simulink model "JFBH"  (Simulink 5.0)
settings: Solver=ode4  StartTime=0.0  StopTime=1  FixedStep=0.001  RelTol=1e-3
settings Model: LastModifiedBy=ThinkPad  RTWOptions="-aEnforceIntegerDowncast=1 -aExtMode=0 -aExtModeTesting=0 -aFoldNonRolledExpr=1 -aForceParamTrailComments=0 -aGenerateComments=1 -aGenerateReport=0 -aIgnoreCustomStorageClasses=1 -aIncDataTypeInIds=0 -aIncHierarchyInIds=0 -aInlineInvariantSignals=0 -aInlinedPrmAccess=\"Literals\" -aLocalBlockOutputs=1 -aLogVarNameModifier=\"rt_\" -aMaxRTWIdLen=31 -aPrefixModelToSubsysFcnNames=1 -aRTWVerbose=1 -aRollThreshold=5 -aShowEliminatedStatements=0"

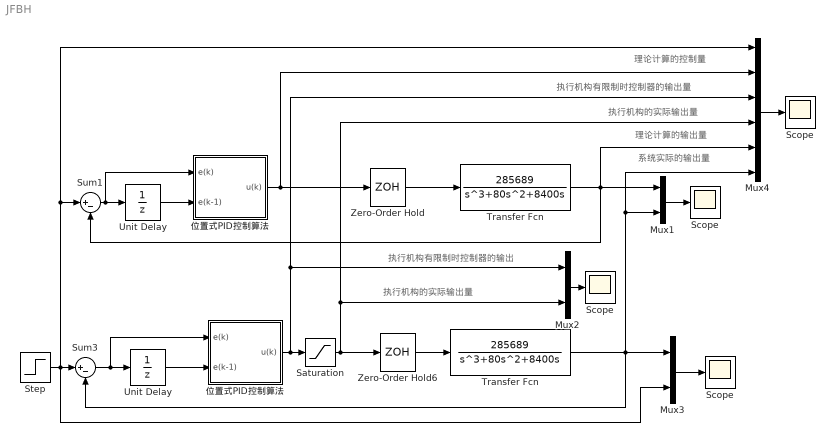
== system JFBH ==
  note: 执行机构有限制时控制器的输出
  note: 执行机构的实际输出量
  note: 执行机构有限制时控制器的输出量
  note: 执行机构的实际输出量
  note: 系统实际的输出量
  note: 理论计算的控制量
  note: 理论计算的输出量
  " Scope " : Scope
      settings: YMin=0  YMax=45  MaxDataPoints=500000
  Mux1 : Mux  Inputs=2
  Mux2 : Mux  Inputs=2
  Mux3 : Mux  Inputs=2
  Mux4 : Mux  Inputs=6
  Saturation : Saturate  UpperLimit=6  LowerLimit=-6
  Scope : Scope
      settings: YMin=0  YMax=45  SaveName=ScopeData6  MaxDataPoints=500000
  "Scope " : Scope
      settings: YMin=0  YMax=45  MaxDataPoints=500000
  "Scope  " : Scope
      settings: YMin=0  YMax=45  SaveName=JFBH  DataFormat=Array  MaxDataPoints=500000
  Step : Step  Time=0  After=30  SampleTime=0
  Sum1 : Sum  Inputs=|+-  SaturateOnIntegerOverflow=on
  Sum3 : Sum  Inputs=|+-  SaturateOnIntegerOverflow=on
  "Transfer Fcn " : TransferFcn  Numerator=[285689]  Denominator="[1 80  8400 0]"
  "Transfer Fcn  " : TransferFcn  Numerator=[285689]  Denominator="[1 80  8400 0]"
  "Unit Delay " : UnitDelay  SampleTime=0.001
  "Unit Delay  " : UnitDelay  SampleTime=0.001
  "Zero-Order Hold  " : ZeroOrderHold  SampleTime=0.001
  Zero-Order Hold6 : ZeroOrderHold  SampleTime=0.001
  "位置式PID控制算法 " : Subsystem
  "位置式PID控制算法  " : Subsystem
  wires:
  "位置式PID控制算法  "/1(u(k)) -> Saturation/1, Mux2/1, Mux4/3
  Zero-Order Hold6/1 -> "Transfer Fcn  "/1
  "Transfer Fcn  "/1 -> Mux3/1, Mux1/2, Mux4/6, Sum3/2
  "Unit Delay  "/1 -> "位置式PID控制算法  "/2(e(k-1))
  Sum3/1 -> "Unit Delay  "/1, "位置式PID控制算法  "/1(e(k))
  Mux3/1 -> Scope/1
  Step/1 -> Sum3/1, Sum1/1, Mux4/1, Mux3/2
  "位置式PID控制算法 "/1(u(k)) -> "Zero-Order Hold  "/1, Mux4/2
  "Zero-Order Hold  "/1 -> "Transfer Fcn "/1
  "Transfer Fcn "/1 -> Mux1/1, Sum1/2, Mux4/5
  "Unit Delay "/1 -> "位置式PID控制算法 "/2(e(k-1))
  Sum1/1 -> "位置式PID控制算法 "/1(e(k)), "Unit Delay "/1
  Mux1/1 -> "Scope "/1
  Mux2/1 -> " Scope "/1
  Saturation/1 -> Zero-Order Hold6/1, Mux2/2, Mux4/4
  Mux4/1 -> "Scope  "/1

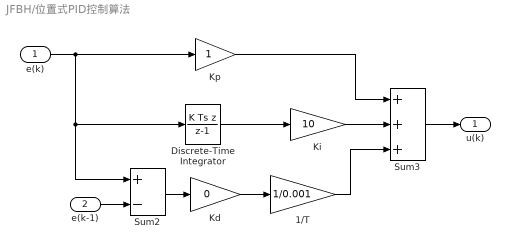
== system JFBH/位置式PID控制算法  ==
  e(k) : Inport
  e(k-1) : Inport  Port=2
  1/T : Gain  Gain=1/0.001  SaturateOnIntegerOverflow=on
  Discrete-Time Integrator : DiscreteIntegrator  IntegratorMethod=Backward Euler  SampleTime=0.001
  Kd : Gain  Gain=0  SaturateOnIntegerOverflow=on
  Ki : Gain  Gain=10  SaturateOnIntegerOverflow=on
  Kp : Gain  SaturateOnIntegerOverflow=on
  Sum2 : Sum  Inputs=+-  SaturateOnIntegerOverflow=on
  Sum3 : Sum  Inputs=+++  SaturateOnIntegerOverflow=on
  u(k) : Outport
  wires:
  Sum2/1 -> Kd/1
  e(k)/1 -> Kp/1, Discrete-Time Integrator/1, Sum2/1
  Kp/1 -> Sum3/1
  Sum3/1 -> u(k)/1
  Kd/1 -> 1/T/1
  Discrete-Time Integrator/1 -> Ki/1
  e(k-1)/1 -> Sum2/2
  1/T/1 -> Sum3/3
  Ki/1 -> Sum3/2

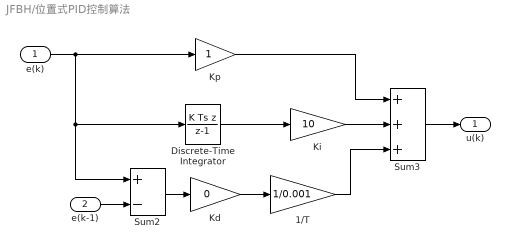
== system JFBH/位置式PID控制算法   ==
  e(k) : Inport
  e(k-1) : Inport  Port=2
  1/T : Gain  Gain=1/0.001  SaturateOnIntegerOverflow=on
  Discrete-Time Integrator : DiscreteIntegrator  IntegratorMethod=Backward Euler  SampleTime=0.001
  Kd : Gain  Gain=0  SaturateOnIntegerOverflow=on
  Ki : Gain  Gain=10  SaturateOnIntegerOverflow=on
  Kp : Gain  SaturateOnIntegerOverflow=on
  Sum2 : Sum  Inputs=+-  SaturateOnIntegerOverflow=on
  Sum3 : Sum  Inputs=+++  SaturateOnIntegerOverflow=on
  u(k) : Outport
  wires:
  Ki/1 -> Sum3/2
  1/T/1 -> Sum3/3
  e(k-1)/1 -> Sum2/2
  Discrete-Time Integrator/1 -> Ki/1
  Kd/1 -> 1/T/1
  Sum3/1 -> u(k)/1
  Kp/1 -> Sum3/1
  e(k)/1 -> Sum2/1, Discrete-Time Integrator/1, Kp/1
  Sum2/1 -> Kd/1
